simulink model "Cascade_Realization"  (R2020b)
settings: Solver=FixedStepDiscrete  StartTime=0.0  StopTime=10.0  FixedStep=1  RelTol=1e-3
settings Model: Creator=Diwakar Reddy  LastModifiedBy=Diwakar Reddy
settings DataIOCC: SaveOutput=off  SaveTime=off

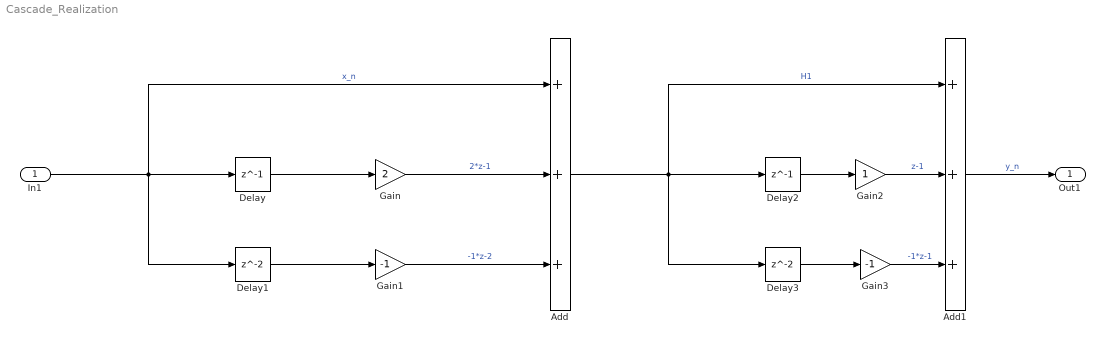
== system Cascade_Realization ==
  In1 : Inport  OutDataTypeStr=double  PortDimensions=[1 1]  SampleTime=[1,0]
  Add : Sum  Inputs=+++
  Add1 : Sum  Inputs=+++
  Delay : Delay  DelayLength=1
  Delay1 : Delay
  Delay2 : Delay  DelayLength=1
  Delay3 : Delay
  Gain : Gain  Gain=2
  Gain1 : Gain  Gain=-1
  Gain2 : Gain
  Gain3 : Gain  Gain=-1
  Out1 : Outport  OutDataTypeStr=double  PortDimensions=[1 1]  SampleTime=[1,0]
  wires:
  Delay/1 -> Gain/1
  Gain/1 -> Add/2  "2*z-1"
  Delay1/1 -> Gain1/1
  Add/1 -> Delay3/1, Delay2/1, Add1/1  "H1"
  In1/1 -> Delay/1, Add/1, Delay1/1  "x_n"
  Delay3/1 -> Gain3/1
  Gain2/1 -> Add1/2  "z-1"
  Gain1/1 -> Add/3  "-1*z-2"
  Gain3/1 -> Add1/3  "-1*z-1"
  Delay2/1 -> Gain2/1
  Add1/1 -> Out1/1  "y_n"
